simulink model "Sequence_Recognizer"  (R2016a)
settings: Solver=FixedStepAuto  StartTime=0.0  StopTime=20.0  FixedStep=1.0  RelTol=1e-3
undefined symbols (not defined in the file or in its folder): sigbuilder_block
settings Model: Creator=SHABBIR  LastModifiedBy=SHABBIR

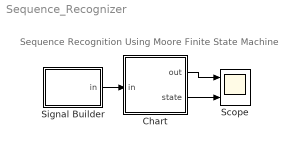
== system Sequence_Recognizer ==
  note: Sequence Recognition Using Moore Finite State Machine
  Chart : Stateflow chart  TreatAsAtomicUnit=on
  Scope : Scope  NumInputPorts=2
  Signal Builder : Subsystem  Tag=STV Subsys  LoadFcn=sigbuilder_block('load');  StartFcn=sigbuilder_block('start');  StopFcn=sigbuilder_block('stop');  ClipboardFcn=sigbuilder_block('clipboard');  mask(Sigbuilder block){}
      mask help: Simulink:masks:SigbuilderBlock_MD
      mask init:
      | if ~strcmp(get_param(bdroot(gcbh),'SimulationStatus'),'stopped') tuvar = sigbuilder_block('maskInit'); end
      settings: CopyFcn=sigbuilder_block('copy');  DeleteFcn=sigbuilder_block('delete');  ModelCloseFcn=sigbuilder_block('modelClose');  PreSaveFcn=sigbuilder_block('preSave');  PauseFcn=sigbuilder_block('pause');  ContinueFcn=sigbuilder_block('continue');  NameChangeFcn=sigbuilder_block('namechange');  OpenFcn=sigbuilder_block('open',[0.75 302.25 510.75 210 ]);  CloseFcn=sigbuilder_block('close');
      mask Display: plot(0, 0, 100, 100,[2, 2, 32, 32, 2], [68, 8, 8, 68, 68],[32, 2], [38, 38], [32, 19, 2],[53, 60, 44], [32, 17, 17, 2],[16, 16, 31, 31]);txt = getActiveGroup(gcbh);text(2, 100, txt,'verticalAlignment', 'top');
  wires:
  Chart/2(state) -> Scope/2
  Chart/1(out) -> Scope/1
  Signal Builder/1(in) -> Chart/1(in)

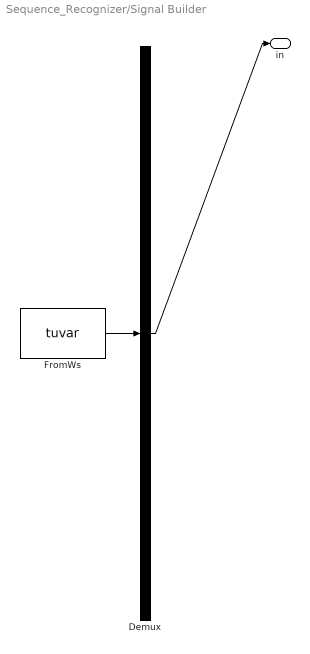
== system Sequence_Recognizer/Signal Builder ==
  Demux : Demux  Tag=STV Demux  Outputs=1
  FromWs : FromWorkspace  Tag=STV FromWs  VariableName=tuvar  SampleTime=0
      SigBuilderData=|
      | common.afterFinalStr = 'Extrapolate'
      | common.sampleTime = 0
      | dataSet.timeRange = [0 20]
      | dataSet.name = 'Group 1'
      | sbobj.Groups.Name = 'Group 1'
      | sbobj.Groups.Signals.Name = 'in'
      | sbobj.Groups.Signals.XData = [0 1 2 2 3 3 4 4 5 5 6 7 8 8 9 10 11 12 12 13 13 14 14 15 15 16 16 17 18 19 19 20]
      | sbobj.Groups.Signals.YData = [0 0 0 1 1 0 0 1 1 0 0 0 0 1 1 1 1 1 0 0 1 1 0 0 1 1 0 0 0 0 1 1]
      | sbobj.Groups.TimeRange = [0 20]
  in : Outport  Tag=STV Outport
  wires:
  FromWs/1 -> Demux/1
  Demux/1 -> in/1

== stateflow chart Sequence_Recognizer/Chart ==
  settings: stateMachineType=MOORE_MACHINE
  state State0
    state=0;
    out=0;
  state State1
    state=1;
    out=0;
  state State10
    state=2;
    out=0;
  state State11
    state=3;
    out=1;
  State11 -> State0 [order 2] : [in==0]
  State11 -> State1 [order 1] : [in==1]
  (default) -> State0
  State0 -> State0 [order 2] : [in==0]
  State1 -> State1 [order 2] : [in==1]
  State0 -> State1 [order 1] : [in==1]
  State1 -> State10 [order 1] : [in==0]
  State10 -> State11 [order 1] : [in==1]
  State10 -> State0 [order 2] : [in==0]
  data: in input; out output double; state output double
